simulink model "transfer_fncs"  (R2023a)
settings: Solver=VariableStepAuto  StartTime=0.0  StopTime=30  RelTol=1e-3
values from neighbouring files (symbols this model uses):
  a1 = Gz.Numerator{1}(2)    [zad1.m]
  a2 = Gz.Numerator{1}(3)    [zad1.m]
  a3 = Gz.Numerator{1}(4)    [zad1.m]
  b0 = Gz.Denominator{1}(1)    [zad1.m]
  b1 = Gz.Denominator{1}(2)    [zad1.m]
  b2 = Gz.Denominator{1}(3)    [zad1.m]
  b3 = Gz.Denominator{1}(4)    [zad1.m]
  T = 0.5    [zad1.m]
settings Model: Creator=denys  LastModifiedBy=denys

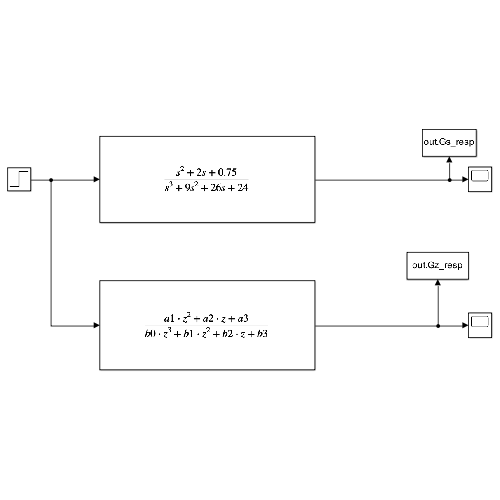
[thumbnail: Simulink's stored preview of the top-level diagram]
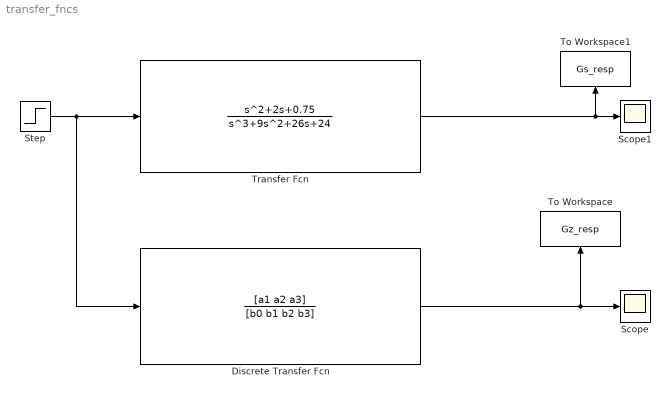
== system transfer_fncs ==
  Discrete Transfer Fcn : DiscreteTransferFcn  Numerator=[a1 a2 a3]  Denominator=[b0 b1 b2 b3]
  Scope : Scope
  Scope1 : Scope
  Step : Step
  To Workspace : ToWorkspace  VariableName=Gz_resp  SaveFormat=Timeseries  SampleTime=T
  To Workspace1 : ToWorkspace  VariableName=Gs_resp  SaveFormat=Timeseries  SampleTime=-1
  Transfer Fcn : TransferFcn  Numerator=[1 2 0.75]  Denominator=[1 9 26 24]
  wires:
  Step/1 -> Discrete Transfer Fcn/1, Transfer Fcn/1
  Transfer Fcn/1 -> To Workspace1/1, Scope1/1
  Discrete Transfer Fcn/1 -> Scope/1, To Workspace/1
